simulink model "EchoUsingWav"  (Simulink 6.5)
settings: Solver=ode45  StartTime=0.0  StopTime=10.0  RelTol=1e-3
libraries: dspwin32 x2, dspsigops x1
settings Model: Creator=Administrator  LastModifiedBy=Administrator

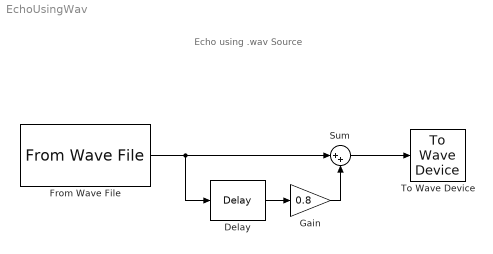
== system EchoUsingWav ==
  note: Echo using .wav Source
  Delay : dspsigops/Delay  dly_unit=Samples  delay=4000  ic_detail=off  dif_ic_for_ch=off  dif_ic_for_dly=off  ic=0  reset_popup=None
  From Wave File : dspwin32/From Wave File  FileName=speech_dft.wav  SamplesPerFrame=256  MinBufSize=256  dType=double  bLoop=off  timesToPlay=1  restartMode=immediately after last sample  firstSampleOutput=off  lastSampleOutput=off
  Gain : Gain  Gain=0.8
  Sum : Sum  Inputs=|++
  To Wave Device : dspwin32/To Wave Device  bufDuration=2  determineBufSize=on  userIntBufSize=256  initDelay=0.1  useDefaultDevice=on  userDeviceID=VIA AC'97 Enhanced Audio (WAVE)  enable24Bit=off
  wires:
  From Wave File/1 -> Sum/1, Delay/1
  Sum/1 -> To Wave Device/1
  Gain/1 -> Sum/2
  Delay/1 -> Gain/1
